simulink library "tqr"  (R2021b)
settings: Solver=VariableStepAuto  StartTime=0.0  StopTime=10.0  RelTol=1e-3
undefined symbols (not defined in the file or in its folder): ATQR_AltRDCActiveFEDUInc_X_pct, ATQR_AltRDCActiveFEDUInc_Y_enum, ATQR_AltRDCActiveFEDUTs_X_pct, ATQR_AltRDCActiveFEDUTs_Y_enum, ATQR_AltRDCActiveREDUInc_X_pct, ATQR_AltRDCActiveREDUInc_Y_enum, ATQR_AltRDCActiveREDUTs_X_pct, ATQR_AltRDCActiveREDUTs_Y_enum, ATQR_CreepFEDUTqIncSR_X_rpm, ATQR_CreepFEDUTqIncSR_Y_Nm, ATQR_CreepFEDUTs_X_rpm, ATQR_CreepFEDUTs_Y_Nm, ATQR_EcoTqFrIncGain_X_Nm, ATQR_EcoTqFrIncGain_Y_pct, ATQR_EcoTqRrIncGain_X_Nm, ATQR_EcoTqRrIncGain_Y_pct, ATQR_EL1FEDUTqDecSR_Y_Nm, ATQR_EL1FEDUTqIncSR_X_rpm, ATQR_EL1FEDUTqIncSR_Y_pct, ATQR_EL1FEDUTs_X_rpm, ATQR_EL1FEDUTs_Y_Nm, ATQR_EL1REDUTqDecSR_Y_Nm, ATQR_EL1REDUTs_Y_Nm, ATQR_FEDUEL1RegenTs_X_rpm, ATQR_FEDUTIPOutTs_X_rpm, ATQR_FrNegRateLimitIncN_X_rpm, ATQR_FrNegRateLimitIncN_Y_Nm, ATQR_FrPosRateLimitIncN_X_rpm, ATQR_FrPosRateLimitIncN_Y_Nm, ATQR_FShaftSpdTqLimCoe_X_rpm, ATQR_FTimerTqLimCoe_X_s, ATQR_FTqZeroTransUpBoundN_X_rpm, ATQR_NL1FEDUTqDecSR_Y_Nm, ATQR_NL1FEDUTqIncSR_X_rpm, ATQR_NL1FEDUTqIncSR_Y_pct, ATQR_NL1FEDUTs_X_rpm, ATQR_NL1FEDUTs_Y_Nm, ATQR_NL1REDUTqDecSR_Y_Nm, ATQR_NL1REDUTs_Y_Nm, ATQR_NormalTqFrIncGain_X_Nm, ATQR_NormalTqFrIncGain_Y_pct, ATQR_NormalTqRrIncGain_X_Nm, ATQR_NormalTqRrIncGain_Y_pct, ATQR_RrNegRateLimitIncN_X_rpm, ATQR_RrNegRateLimitIncN_Y_Nm, ATQR_RrPosRateLimitIncN_X_rpm, ATQR_RrPosRateLimitIncN_Y_Nm, ATQR_RShaftSpdTqLimCoe_X_rpm, ATQR_RTimerTqLimCoe_X_s, ATQR_SL1FEDUTqDecSR_Y_Nm, ATQR_SL1FEDUTqIncSR_X_rpm, ATQR_SL1FEDUTqIncSR_Y_pct, ATQR_SL1FEDUTs_X_rpm, ATQR_SL1FEDUTs_Y_Nm, ATQR_SL1REDUTqDecSR_Y_Nm, ATQR_SL1REDUTs_Y_Nm, ATQR_SportTqFrIncGain_X_Nm, ATQR_SportTqFrIncGain_Y_pct, ATQR_SportTqRrIncGain_X_Nm, ATQR_SportTqRrIncGain_Y_pct ... (+261)
libraries: hcu_lib x14, simulink x12, $bdroot x3
(part 2 of 9)

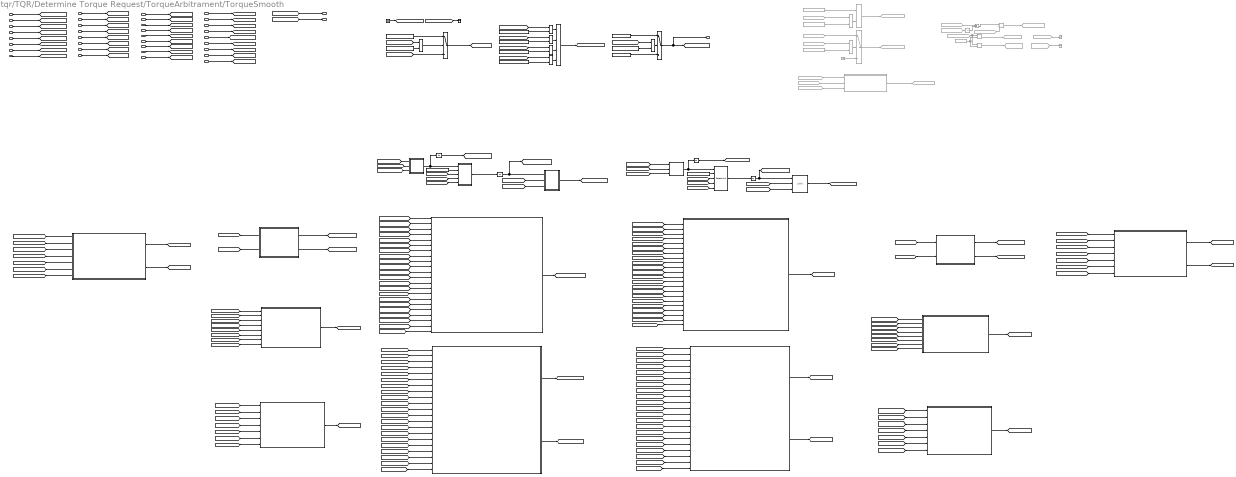
== system tqr/TQR/Determine Torque Request/TorqueArbitrament/TorqueSmooth ==
  note: Fr | Rr
  note: Front First order filter input tau map and determination
  note: Rear Rate limitation map and determination
  note: Front Rate limitation map and determination
  note: Rear wheel first order filter input torque command determination
  note: Front wheel first order filter input torque command determination:
  note: Rear Torque zero point transfer status determination
  note: Front Torque zero point transfer status determination
  note: Front Torque zero point transfer boundary map
  note: Rear Torque zero point transfer boundary map
  note: Rear First order filter input tau map and determination
  note: Rear torque ramp limtation and determination
  note: Rear torque ramp limtation and determination
  note: Rear Final Torque
  note: Front Final Torque
  task_time_s : Inport
  VDHP_ActAPSPosn_pct : Inport  Port=2
  VTQD_TqTargetShaftSpd_rpm : Inport  Port=3
  VTQD_TqSourceFr_enum : Inport  Port=4
  VTQD_TqSourceRr_enum : Inport  Port=5
  VTQD_AfterAvailableTqDemRr_Nm : Inport  Port=6
  VTQD_AfterAvailableTqDemFr_Nm : Inport  Port=7
  VTQD_EVDriveMode_enum : Inport  Port=8
  VTQD_EVDriveModeValid_flg : Inport  Port=9
  VTQD_RollRegenEnable_flg : Inport  Port=10
  VINP_VehSpeed_kph : Inport  Port=11
  VPMM_DriveTrainSelect_enum : Inport  Port=12
  VTQD_LimpHomeAct_flg : Inport  Port=13
  VTQD_RegenMode_enum : Inport  Port=14
  VVMC_ACCPedalOvrd_flg : Inport  Port=15
  VVMC_CCPedalOvrd_flg : Inport  Port=16
  VTQD_GearActualPosn_enum : Inport  Port=17
  VTQD_PreLoadHold_flg : Inport  Port=18
  VTQD_PreLoadPreEn_flg : Inport  Port=19
  VTQR_NoABSFEDUWhlTqReq_Nm : Inport  Port=20
  VTQR_NoABSREDUWhlTqReq_Nm : Inport  Port=21
  VTQD_CreepPrLoadEnable_flg : Inport  Port=22
  VVMC_ADASActive_flg : Inport  Port=23
  VTQD_RDCActive_enum : Inport  Port=24
  VVMC_ActMaxSlideRate_pct : Inport  Port=25
  VTQD_RegenTqLimitEn_flg : Inport  Port=26
  VTQD_PedAccTqEn_flg : Inport  Port=27
  VTQR_FrGearChange_flg : Inport  Port=28
  VTQR_RrGearChange_flg : Inport  Port=29
  VVMC_MSAWhlTqActive_flg : Inport  Port=30
  VINP_LFRawWhlSpeed_kph : Inport  Port=31
  VINP_RFRawWhlSpeed_kph : Inport  Port=32
  VINP_LRRawWhlSpeed_kph : Inport  Port=33
  VINP_RRRawWhlSpeed_kph : Inport  Port=34
  AND : Logic  Inputs=4  AllPortsSameDT=off  OutDataTypeStr=boolean
  AND18 : Logic  Commented=on  AllPortsSameDT=off  OutDataTypeStr=boolean
  Constant : Constant  Value=ZERO_FLOAT
  Constant1 : Constant  Value=ZERO_FLOAT
  Constant2 : Constant  Value=ENUM_REGENLEVEL_LV1
  Constant3 : Constant  Value=MINUSONE_FLOAT
  Constant36 : Constant  Commented=on  Value=KTQR_AWDSynchEnbl_flg
  Constant38 : Constant  Commented=on  Value=ENUM_DRIVETRAIN_AWD
  Constant4 : Constant  Value=ENUM_DRIVEMODE_SPORT
  Constant41 : Constant  Commented=on  Value=ZERO_INT
  Constant47 : Constant  Commented=on  Value=ENUM_DRIVETRAIN_FWD
  Constant5 : Constant  Value=KTQR_LaunchEnPedal_pct
  Constant6 : Constant  Value=KTQR_LaunchEnSpd_kph
  Constant7 : Constant  Value=ONE_FLOAT
  Divide : Product  Commented=on  Inputs=*/
  Equal{,1..3} (4 alike) : RelationalOperator  Operator===  OutDataTypeStr=boolean  RndMeth=Simplest
  Equal34 : RelationalOperator  Commented=on  Operator===  OutDataTypeStr=boolean  RndMeth=Simplest
  Equal35 : RelationalOperator  Commented=on  Operator===  OutDataTypeStr=boolean  RndMeth=Simplest
  FirstOrderFilter : Subsystem  RTWFileName=HCU_LIB  mask(FirstOrderFilter){}
      mask help: First order Filter.
      settings: RTWFileNameOpts=User specified
  FirstOrderFilter1 : $bdroot/TQR/Determine Torque Request/TorqueArbitrament/TorqueSmooth/FirstOrderFilter
  From125 : From  Commented=on  GotoTag=VDHP_ActAPSPosn_pct
  From127 : From  Commented=on  GotoTag=VTQR_ActAPSPosnAcc_enum
  From139 : From  Commented=on  GotoTag=VTQR_PedalAcc_flg
  From140 : From  Commented=on  GotoTag=VTQR_PedalDec_flg
  From141 : From  Commented=on  GotoTag=VDHP_ActAPSPosn_pct
  From142 : From  Commented=on  GotoTag=task_time_s
  From153 : From  Commented=on  GotoTag=VTQD_TqTargetShaftSpd_rpm
  From154 : From  Commented=on  GotoTag=VPMM_DriveTrainSelect_enum
  From155 : From  Commented=on  GotoTag=VPMM_DriveTrainSelect_enum
  From5 : From  Commented=on  GotoTag=VTQD_DRTransfer_flg
      settings: CloseFcn=tagdialog Close
  From6 : From  Commented=on  GotoTag=NTQR_TMTqReq_Nm
      settings: CloseFcn=tagdialog Close
  From9 : From  Commented=on  GotoTag=VTQR_TMTqReqLimit_Nm
      settings: CloseFcn=tagdialog Close
  Front First order filter input tau map and determination : Subsystem
  Front Torque zero point transfer boundary map : Subsystem
  "Front Torque zero point transfer status determination " : Subsystem
  Front torque ramp limtation and determination : Subsystem
  Front wheel first order filter input torque command determination : Subsystem
  Front wheel rate limit determination : Subsystem
  Goto19 : Goto  Commented=on  GotoTag=VTQR_AWDSynchEnbl_flg
  Goto2 : Goto  Commented=on  GotoTag=VTQR_ZeroTqRecover_flg
  Goto22 : Goto  Commented=on  GotoTag=VTQR_ActAPSPosnAcc_enum
  Goto23 : Goto  Commented=on  GotoTag=VTQR_PedalAcc_flg
  Goto24 : Goto  Commented=on  GotoTag=VTQR_PedalDec_flg
  Goto9 : Goto  Commented=on  GotoTag=VTQD_CAN2TqTargetShaftSpd_rpm
  GreaterThan : RelationalOperator  Commented=on  Operator=>  OutDataTypeStr=boolean  RndMeth=Simplest
  Ground : Ground  Commented=on
  Ground1 : Ground
  Less Than : RelationalOperator  Commented=on  Operator=<  OutDataTypeStr=boolean  RndMeth=Simplest
  Limit : Subsystem  RTWFileName=HCU_LIB  mask(Limit){}
      mask help: Limit funcion.
      settings: RTWFileNameOpts=User specified
  Limit2 : $bdroot/TQR/Determine Torque Request/TorqueArbitrament/TorqueSmooth/Limit
  RateLimit : Subsystem  RTWFileName=HCU_LIB  mask(RateLimit){}
      mask help: Rate limit function.
      settings: RTWFileNameOpts=User specified
  RateLimit1 : $bdroot/TQR/Determine Torque Request/TorqueArbitrament/TorqueSmooth/RateLimit
  Rear First order filter input tau map and determination : Subsystem
  Rear Torque zero point transfer boundary map : Subsystem
  "Rear Torque zero point transfer status determination " : Subsystem
  Rear torque ramp limtation and determination : Subsystem
  Rear wheel first order filter input torque command determination : Subsystem
  Rear wheel rate limit determination : Subsystem
  RegenLV_inc1 : Constant  Value=ENUM_GEARACTUALPOSN_R
  RegenLV_inc5 : Constant  Value=ENUM_GEARACTUALPOSN_R
  RegenLV_inc6 : Constant  Value=ENUM_DRIVEMODE_NRM
  Relational Operator4 : RelationalOperator  Operator=>  OutDataTypeStr=boolean  RndMeth=Simplest
  Relational Operator6 : RelationalOperator  Operator=<=  OutDataTypeStr=boolean  RndMeth=Simplest
  Subtract : Sum  Commented=on  Inputs=+-
  Switch : Switch  Criteria=u2 ~= 0
  Switch1 : Switch  Criteria=u2 > Threshold
  Switch10 : Switch  Commented=on  Criteria=u2 ~= 0
      settings: AttributesFormatString=<%<Criteria>>
  Terminator : Terminator  Commented=on
  Terminator1 : Terminator  Commented=on
  Terminator2 : Terminator
  Unit Delay : UnitDelay  Commented=on  SampleTime=-1  HasFrameUpgradeWarning=on
  Unit Delay{1..4} (4 alike) : UnitDelay  SampleTime=-1
  Zero Torque Revert : Subsystem  Commented=on
  VTQR_RampFEDUWhlTqReq_Nm : Outport
  VTQR_RampREDUWhlTqReq_Nm : Outport  Port=2
  VTQR_RampTqCMDGain_c : Outport  Port=3
  wires:
  [task_time_s] -> FirstOrderFilter/2(Tc)
  FirstOrderFilter/1(out) -> Unit Delay3/1, RateLimit/1(input_raw)  "VTQR_FrFirstOrderOutTq_Nm"
  task_time_s/1 -> [task_time_s]
  RateLimit/1(output) -> Unit Delay1/1  "VTQR_FEDUWhlTqReqSmooth_Nm"
  Unit Delay1/1 -> [VTQR_FEDUWhlTqReqSmoothDelay_Nm], Limit/1(input)  "VTQR_FEDUWhlTqReqSmoothDelay_Nm"
  From5/1 -> Zero Torque Revert/1(VTQD_DRTransfer_flg)
  Zero Torque Revert/1(VTQR_ZeroTqRecover_flg) -> Goto2/1
  From6/1 -> Zero Torque Revert/2(NTQR_TMTqReq_Nm)
  From9/1 -> Zero Torque Revert/3(VTQR_TMTqReqLimit_Nm)
  [VTQR_ActFEDUTrqUpLim_Nm] -> Limit/2(upper_limit)
  [VTQR_ActFEDUTrqLowLim_Nm] -> Limit/3(lower_limit)
  Limit/1(out) -> [VTQR_RampFEDUWhlTqReq_Nm]  "VTQR_RampFEDUWhlTqReq_Nm"
  [task_time_s] -> RateLimit/3(steptime)
  Constant/1 -> RateLimit/2(initial_value)
  VTQD_TqSourceFr_enum/1 -> [VTQD_TqSourceFr_enum]
  VDHP_ActAPSPosn_pct/1 -> [VDHP_ActAPSPosn_pct]
  VTQD_AfterAvailableTqDemFr_Nm/1 -> [VTQD_AfterAvailableTqDemFr_Nm]
  VTQD_AfterAvailableTqDemRr_Nm/1 -> [VTQD_AfterAvailableTqDemRr_Nm]
  Unit Delay2/1 -> [VTQR_REDUWhlTqReqSmoothDelay_Nm], Limit2/1  "VTQR_REDUWhlTqReqSmoothDelay_Nm"
  RateLimit1/1 -> Unit Delay2/1  "VTQR_REDUWhlTqReqSmooth_Nm"
  FirstOrderFilter1/1 -> Unit Delay4/1, RateLimit1/1  "VTQR_RrFirstOrderOutTq_Nm"
  [task_time_s] -> FirstOrderFilter1/2
  Limit2/1 -> [VTQR_RampREDUWhlTqReq_Nm]  "VTQR_RampREDUWhlTqReq_Nm"
  [task_time_s] -> RateLimit1/3
  Constant1/1 -> RateLimit1/2
  VTQD_EVDriveMode_enum/1 -> [VTQD_EVDriveMode_enum]
  Constant38/1 -> Equal34/2
  Equal34/1 -> AND18/2
  From154/1 -> Equal34/1
  Constant36/1 -> AND18/1
  AND18/1 -> Goto19/1  "VTQR_AWDSynchEnbl_flg"
  From125/1 -> Subtract/1
  Divide/1 -> Goto22/1  "VTQR_ActAPSPosnAcc_enum"
  From127/1 -> Less Than/1, GreaterThan/1
  Constant41/1 -> Less Than/2, GreaterThan/2
  GreaterThan/1 -> Goto23/1  "VTQR_PedalAcc_flg"
  Less Than/1 -> Goto24/1  "VTQR_PedalDec_flg"
  From139/1 -> Terminator/1
  From140/1 -> Terminator1/1
  From141/1 -> Unit Delay/1
  Unit Delay/1 -> Subtract/2
  Subtract/1 -> Divide/1
  From142/1 -> Divide/2
  VTQD_RollRegenEnable_flg/1 -> [VTQD_RollRegenEnable_flg]
  VINP_VehSpeed_kph/1 -> [VINP_VehSpeed_kph]
  From155/1 -> Equal35/1
  Constant47/1 -> Equal35/2
  Equal35/1 -> Switch10/2
  Switch10/1 -> Goto9/1
  From153/1 -> Switch10/1
  VPMM_DriveTrainSelect_enum/1 -> [VPMM_DriveTrainSelect_enum]
  VTQD_LimpHomeAct_flg/1 -> [VTQD_LimpHomeAct_flg]
  VTQD_EVDriveModeValid_flg/1 -> [VTQD_EVDriveModeValid_flg]
  Ground/1 -> Switch10/3
  VTQD_TqSourceRr_enum/1 -> [VTQD_TqSourceRr_enum]
  [VTQR_FEDUWhlTqReqSmoothDelay_Nm] -> "Front Torque zero point transfer status determination "/1(VTQR_FEDUWhlTqReqSmoothDelay_Nm)
  [VTQR_FrTqZeroTransUpBound_Nm] -> "Front Torque zero point transfer status determination "/2(VTQR_FrTqZeroTransUpBound_Nm)
  [VTQR_FrTqZeroTransLowBound_Nm] -> "Front Torque zero point transfer status determination "/3(VTQR_FrTqZeroTransLowBound_Nm)
  "Front Torque zero point transfer status determination "/1(VTQR_FrTqZeroTrans_enum) -> [VTQR_FrTqZeroTrans_enum]
  Front wheel first order filter input torque command determination/1(VTQR_FrFirstOrderInpTq_Nm) -> [VTQR_FrFirstOrderInpTq_Nm]
  Rear wheel first order filter input torque command determination/1(VTQR_RrFirstOrderInpTq_Nm) -> [VTQR_RrFirstOrderInpTq_Nm]
  [VTQR_FrTqZeroTrans_enum] -> Front wheel rate limit determination/1(VTQR_FrTqZeroTrans_enum)
  [VTQD_TqSourceFr_enum] -> Front wheel rate limit determination/2(VTQD_TqSourceFr_enum)
  [VTQD_TqTargetShaftSpd_rpm] -> Front wheel rate limit determination/3(VTQD_TqTargetShaftSpd_rpm)
  Front wheel rate limit determination/2(VTQR_FrRateLimitDec_Nm) -> [VTQR_FrRateLimitDec_Nm]
  Front wheel rate limit determination/1(VTQR_FrRateLimitInc_Nm) -> [VTQR_FrRateLimitInc_Nm]
  [VTQR_FrFirstOrderInpTq_Nm] -> FirstOrderFilter/1(in)
  [VTQR_RrFirstOrderInpTq_Nm] -> FirstOrderFilter1/1
  [VTQR_FrRateLimitInc_Nm] -> RateLimit/4(ratelimt_inc)
  [VTQR_FrRateLimitDec_Nm] -> RateLimit/5(ratelimt_dec)
  Rear wheel rate limit determination/1(VTQR_RrRateLimitInc_Nm) -> [VTQR_RrRateLimitInc_Nm]
  Rear wheel rate limit determination/2(VTQR_RrRateLimitDec_Nm) -> [VTQR_RrRateLimitDec_Nm]
  [VTQD_TqTargetShaftSpd_rpm] -> Rear wheel rate limit determination/3(VTQD_TqTargetShaftSpd_rpm)
  [VTQD_TqSourceRr_enum] -> Rear wheel rate limit determination/2(VTQD_TqSourceRr_enum)
  [VTQR_RrTqZeroTrans_enum] -> Rear wheel rate limit determination/1(VTQR_RrTqZeroTrans_enum)
  [VTQR_RrRateLimitInc_Nm] -> RateLimit1/4
  [VTQR_RrRateLimitDec_Nm] -> RateLimit1/5
  Unit Delay3/1 -> [VTQR_FrFirstOrderOutTqDelay_Nm]  "VTQR_FrFirstOrderOutTqDelay_Nm"
  Front First order filter input tau map and determination/1(VTQR_FrFirstOrderInpTs_c) -> [VTQR_FrFirstOrderInpTs_c]
  [VTQR_FrFirstOrderInpTs_c] -> FirstOrderFilter/3(Ts)
  Rear First order filter input tau map and determination/1(VTQR_RrFirstOrderInpTs_c) -> [VTQR_RrFirstOrderInpTs_c]
  [VTQR_RrFirstOrderInpTs_c] -> FirstOrderFilter1/3
  Unit Delay4/1 -> [VTQR_RrFirstOrderOutTqDelay_Nm]  "VTQR_RrFirstOrderOutTqDelay_Nm"
  [VTQD_TqTargetShaftSpd_rpm] -> Front First order filter input tau map and determination/1(VTQD_TqTargetShaftSpd_rpm)
  [VTQR_EVDriveMode_enum] -> Front First order filter input tau map and determination/2(VTQR_EVDriveMode_enum)
  [VTQD_RollRegenEnable_flg] -> Front First order filter input tau map and determination/3(VTQD_RollRegenEnable_flg)
  [VTQD_TqSourceFr_enum] -> Front First order filter input tau map and determination/4(VTQD_TqSourceFr_enum)
  [VTQR_FEDUWhlTqReqSmoothDelay_Nm] -> Front First order filter input tau map and determination/5(VTQR_FEDUWhlTqReqSmoothDelay_Nm)
  [VDHP_ActAPSPosn_pct] -> Front First order filter input tau map and determination/6(VDHP_ActAPSPosn_pct)
  [VINP_VehSpeed_kph] -> Front First order filter input tau map and determination/7(VINP_VehSpeed_kph)
  [VTQD_LimpHomeAct_flg] -> Front First order filter input tau map and determination/8(VTQD_LimpHomeAct_flg)
  [VTQD_TqTargetShaftSpd_rpm] -> Rear First order filter input tau map and determination/1(VTQD_TqTargetShaftSpd_rpm)
  [VTQR_EVDriveMode_enum] -> Rear First order filter input tau map and determination/2(VTQR_EVDriveMode_enum)
  [VTQD_RollRegenEnable_flg] -> Rear First order filter input tau map and determination/3(VTQD_RollRegenEnable_flg)
  [VTQD_TqSourceRr_enum] -> Rear First order filter input tau map and determination/4(VTQD_TqSourceRr_enum)
  [VTQR_REDUWhlTqReqSmoothDelay_Nm] -> Rear First order filter input tau map and determination/5(VTQR_REDUWhlTqReqSmooth_Nm)
  [VDHP_ActAPSPosn_pct] -> Rear First order filter input tau map and determination/6(VDHP_ActAPSPosn_pct)
  [VINP_VehSpeed_kph] -> Rear First order filter input tau map and determination/7(VINP_VehSpeed_kph)
  [VTQD_LimpHomeAct_flg] -> Rear First order filter input tau map and determination/8(VTQD_LimpHomeAct_flg)
  [VTQD_LimpHomeAct_flg] -> Front wheel rate limit determination/4(VTQD_LimpHomeAct_flg)
  [VTQR_EVDriveMode_enum] -> Front wheel rate limit determination/5(VTQR_EVDriveMode_enum)
  [VDHP_ActAPSPosn_pct] -> Front wheel rate limit determination/6(VDHP_ActAPSPosn_pct)
  [VTQR_FEDUWhlTqReqSmoothDelay_Nm] -> Front wheel rate limit determination/7(VTQR_FEDUWhlTqReqSmoothDelay_Nm)
  [VTQD_EVDriveModeValid_flg] -> Front wheel rate limit determination/8(VTQD_EVDriveModeValid_flg)
  [VTQD_LimpHomeAct_flg] -> Rear wheel rate limit determination/4(VTQD_LimpHomeAct_flg)
  [VTQR_EVDriveMode_enum] -> Rear wheel rate limit determination/5(VTQR_EVDriveMode_enum)
  [VDHP_ActAPSPosn_pct] -> Rear wheel rate limit determination/6(VDHP_ActAPSPosn_pct)
  [VTQR_REDUWhlTqReqSmoothDelay_Nm] -> Rear wheel rate limit determination/7(VTQR_REDUWhlTqReqSmoothDelay_Nm)
  [VTQD_EVDriveModeValid_flg] -> Rear wheel rate limit determination/8(VTQD_EVDriveModeValid_flg)
  [VTQD_EVDriveModeValid_flg] -> Rear First order filter input tau map and determination/9(VTQD_EVDriveModeValid_flg)
  [VTQD_EVDriveModeValid_flg] -> Front First order filter input tau map and determination/9(VTQD_EVDriveModeValid_flg)
  [VTQD_TqTargetShaftSpd_rpm] -> Front Torque zero point transfer boundary map/1(VTQD_TqTargetShaftSpd_rpm)
  [VTQR_EVDriveMode_enum] -> Front Torque zero point transfer boundary map/2(VTQR_EVDriveMode_enum)
  Front Torque zero point transfer boundary map/1(VTQR_FrTqZeroTransUpBound_Nm) -> [VTQR_FrTqZeroTransUpBound_Nm]
  Front Torque zero point transfer boundary map/2(VTQR_FrTqZeroTransLowBound_Nm) -> [VTQR_FrTqZeroTransLowBound_Nm]
  [VTQD_TqTargetShaftSpd_rpm] -> Rear Torque zero point transfer boundary map/1(VTQD_TqTargetShaftSpd_rpm)
  [VTQR_EVDriveMode_enum] -> Rear Torque zero point transfer boundary map/2(VTQR_EVDriveMode_enum)
  Rear Torque zero point transfer boundary map/1(VTQR_RrTqZeroTransUpBound_Nm) -> [VTQR_RrTqZeroTransUpBound_Nm]
  Rear Torque zero point transfer boundary map/2(VTQR_RrTqZeroTransLowBound_Nm) -> [VTQR_RrTqZeroTransLowBound_Nm]
  [VTQD_RegenMode_enum] -> Front First order filter input tau map and determination/10(VTQD_RegenMode_enum)
  VTQD_RegenMode_enum/1 -> [VTQD_RegenMode_enum]
  [VTQD_RegenMode_enum] -> Front wheel rate limit determination/9(VTQD_RegenMode_enum)
  [VTQD_RegenMode_enum] -> Rear First order filter input tau map and determination/10(VTQD_RegenMode_enum)
  [VTQD_RegenMode_enum] -> Rear wheel rate limit determination/9(VTQD_RegenMode_enum)
  VVMC_ACCPedalOvrd_flg/1 -> [VVMC_ACCPedalOvrd_flg]
  VVMC_CCPedalOvrd_flg/1 -> [VVMC_CCPedalOvrd_flg]
  RegenLV_inc5/1 -> Equal/2
  Equal/1 -> Switch/2
  RegenLV_inc6/1 -> Switch/1
  Switch/1 -> [VTQR_EVDriveMode_enum]  "VTQR_EVDriveMode_enum"
  [VTQD_GearActualPosn_enum] -> Equal/1
  [VTQD_EVDriveMode_enum] -> Switch/3
  VTQD_GearActualPosn_enum/1 -> [VTQD_GearActualPosn_enum]
  [VVMC_ACCPedalOvrd_flg] -> Front First order filter input tau map and determination/11(VVMC_ACCPedalOvrd_flg)
  [VVMC_CCPedalOvrd_flg] -> Front First order filter input tau map and determination/12(VVMC_CCPedalOvrd_flg)
  [VVMC_ACCPedalOvrd_flg] -> Front wheel rate limit determination/10(VVMC_ACCPedalOvrd_flg)
  [VVMC_CCPedalOvrd_flg] -> Front wheel rate limit determination/11(VVMC_CCPedalOvrd_flg)
  [VVMC_ACCPedalOvrd_flg] -> Rear First order filter input tau map and determination/11(VVMC_ACCPedalOvrd_flg)
  [VVMC_CCPedalOvrd_flg] -> Rear First order filter input tau map and determination/12(VVMC_CCPedalOvrd_flg)
  [VVMC_ACCPedalOvrd_flg] -> Rear wheel rate limit determination/10(VVMC_ACCPedalOvrd_flg)
  [VVMC_CCPedalOvrd_flg] -> Rear wheel rate limit determination/11(VVMC_CCPedalOvrd_flg)
  VTQD_TqTargetShaftSpd_rpm/1 -> [VTQD_TqTargetShaftSpd_rpm]
  VTQD_PreLoadHold_flg/1 -> [VTQD_PreLoadHold_flg]
  VTQD_PreLoadPreEn_flg/1 -> [VTQD_PreLoadPreEn_flg]
  [VTQD_PreLoadHold_flg] -> Rear First order filter input tau map and determination/13(VTQD_PreLoadHold_flg)
  [VTQD_PreLoadHold_flg] -> Front First order filter input tau map and determination/13(VTQD_PreLoadHold_flg)
  VTQR_NoABSFEDUWhlTqReq_Nm/1 -> [VTQR_NoABSFEDUWhlTqReq_Nm]
  VTQR_NoABSREDUWhlTqReq_Nm/1 -> [VTQR_NoABSREDUWhlTqReq_Nm]
  VTQD_CreepPrLoadEnable_flg/1 -> [VTQD_CreepPrLoadEnable_flg]
  VVMC_ADASActive_flg/1 -> [VVMC_ADASActive_flg]
  [VTQD_CreepPrLoadEnable_flg] -> "Front Torque zero point transfer status determination "/4(VTQD_CreepPrLoadEnable_flg)
  [VVMC_ADASActive_flg] -> "Front Torque zero point transfer status determination "/5(VVMC_ADASActive_flg)
  [VTQD_PreLoadPreEn_flg] -> "Front Torque zero point transfer status determination "/6(VTQD_PreLoadPreEn_flg)
  [VTQD_CreepPrLoadEnable_flg] -> Front First order filter input tau map and determination/15(VTQD_CreepPrLoadEnable_flg)
  [VTQD_CreepPrLoadEnable_flg] -> Rear First order filter input tau map and determination/15(VTQD_CreepPrLoadEnable_flg)
  [VTQD_CreepPrLoadEnable_flg] -> Front wheel rate limit determination/12(VTQD_CreepPrLoadEnable_flg)
  [VTQD_RDCActive_enum] -> Front wheel rate limit determination/14(VTQD_RDCActive_enum)
  [VTQD_PreLoadPreEn_flg] -> Front wheel rate limit determination/15(VTQD_PreLoadPreEn_flg)
  VTQD_RDCActive_enum/1 -> [VTQD_RDCActive_enum]
  [VTQD_PreLoadPreEn_flg] -> Rear wheel rate limit determination/15(VTQD_PreLoadPreEn_flg)
  [VTQD_CreepPrLoadEnable_flg] -> Rear wheel rate limit determination/12(VTQD_CreepPrLoadEnable_flg)
  [VTQD_RDCActive_enum] -> Rear wheel rate limit determination/14(VTQD_RDCActive_enum)
  Ground1/1 -> [VINP_SCPSystemMode_enum]
  [VTQD_RDCActive_enum] -> Front First order filter input tau map and determination/16(VTQD_RDCActive_enum)
  [VTQR_NoABSFEDUWhlTqReq_Nm] -> Front First order filter input tau map and determination/17(VTQR_NoABSFEDUWhlTqReq_Nm)
  [VTQR_RampFEDUWhlTqReq_Nm] -> Front First order filter input tau map and determination/18(VTQR_RampFEDUWhlTqReq_Nm)
  [VTQR_NoABSFEDUWhlTqReq_Nm] -> Front wheel rate limit determination/16(VTQR_NoABSFEDUWhlTqReq_Nm)
  [VTQR_RampFEDUWhlTqReq_Nm] -> Front wheel rate limit determination/17(VTQR_RampFEDUWhlTqReq_Nm)
  [VTQD_RDCActive_enum] -> Rear First order filter input tau map and determination/16(VTQD_RDCActive_enum)
  [VTQR_NoABSREDUWhlTqReq_Nm] -> Rear First order filter input tau map and determination/17(VTQR_NoABSREDUWhlTqReq_Nm)
  [VTQR_RampREDUWhlTqReq_Nm] -> Rear First order filter input tau map and determination/18(VTQR_RampREDUWhlTqReq_Nm)
  [VTQR_NoABSREDUWhlTqReq_Nm] -> Rear wheel rate limit determination/16(VTQR_NoABSREDUWhlTqReq_Nm)
  [VTQR_RampREDUWhlTqReq_Nm] -> Rear wheel rate limit determination/17(VTQR_RampREDUWhlTqReq_Nm)
  [VTQR_FrFirstOrderInpTq_Nm] -> Front First order filter input tau map and determination/19(VTQR_FrFirstOrderInpTq_Nm)
  [VTQR_FrFirstOrderInpTq_Nm] -> Front wheel rate limit determination/18(VTQR_FrFirstOrderInpTq_Nm)
  [VTQR_RrFirstOrderInpTq_Nm] -> Rear First order filter input tau map and determination/19(VTQR_RrFirstOrderInpTq_Nm)
  [VTQR_RrFirstOrderInpTq_Nm] -> Rear wheel rate limit determination/18(VTQR_RrFirstOrderInpTq_Nm)
  [VTQR_ActREDUTrqUpLim_Nm] -> Limit2/2
  [VTQR_ActREDUTrqLowLim_Nm] -> Limit2/3
  VVMC_ActMaxSlideRate_pct/1 -> [VVMC_ActMaxSlideRate_pct]
  VTQD_RegenTqLimitEn_flg/1 -> [VTQD_RegenTqLimitEn_flg]
  VTQD_PedAccTqEn_flg/1 -> [VTQD_PedAccTqEn_flg]
  [VVMC_ActMaxSlideRate_pct] -> Front First order filter input tau map and determination/14(VVMC_ActMaxSlideRate_pct)
  [VVMC_ActMaxSlideRate_pct] -> Front wheel rate limit determination/19(VVMC_ActMaxSlideRate_pct)
  [VTQD_PedAccTqEn_flg] -> Front wheel rate limit determination/20(VTQD_PedAccTqEn_flg)
  [VTQD_RegenTqLimitEn_flg] -> Front wheel rate limit determination/13(VTQD_RegenTqLimitEn_flg)
  [VTQD_PedAccTqEn_flg] -> Rear wheel rate limit determination/20(VTQD_PedAccTqEn_flg)
  [VVMC_ActMaxSlideRate_pct] -> Rear wheel rate limit determination/19(VVMC_ActMaxSlideRate_pct)
  [VVMC_ActMaxSlideRate_pct] -> Rear First order filter input tau map and determination/14(VVMC_ActMaxSlideRate_pct)
  [VTQD_PedAccTqEn_flg] -> Rear First order filter input tau map and determination/20(VTQD_PedAccTqEn_flg)
  Constant5/1 -> Relational Operator4/2
  Relational Operator4/1 -> AND/1
  Equal2/1 -> AND/4
  [VTQR_EVDriveMode_enum] -> Equal1/1
  Equal1/1 -> AND/3
  [VDHP_ActAPSPosn_pct] -> Relational Operator4/1
  [VINP_VehSpeed_kph] -> Relational Operator6/1
  Relational Operator6/1 -> AND/2
  AND/1 -> [VTQR_LaunchEn_flg]  "VTQR_LaunchEn_flg"
  [VTQD_RegenMode_enum] -> Equal2/1
  Constant6/1 -> Relational Operator6/2
  Constant2/1 -> Equal2/2
  Constant4/1 -> Equal1/2
  [VTQR_LaunchEn_flg] -> "Front Torque zero point transfer status determination "/7(VTQR_LaunchEn_flg)
  [VVMC_ACCPedalOvrd_flg] -> "Front Torque zero point transfer status determination "/8(VVMC_ACCPedalOvrd_flg)
  [VTQR_LaunchEn_flg] -> "Rear Torque zero point transfer status determination "/7(VTQR_LaunchEn_flg)
  [VTQD_CreepPrLoadEnable_flg] -> "Rear Torque zero point transfer status determination "/4(VTQD_CreepPrLoadEnable_flg)
  "Rear Torque zero point transfer status determination "/1(VTQR_RrTqZeroTrans_enum) -> [VTQR_RrTqZeroTrans_enum]
  [VVMC_ADASActive_flg] -> "Rear Torque zero point transfer status determination "/5(VVMC_ADASActive_flg)
  [VTQD_PreLoadPreEn_flg] -> "Rear Torque zero point transfer status determination "/6(VTQD_PreLoadPreEn_flg)
  [VTQR_REDUWhlTqReqSmoothDelay_Nm] -> "Rear Torque zero point transfer status determination "/1(VTQR_REDUWhlTqReqSmoothDelay_Nm)
  [VVMC_ACCPedalOvrd_flg] -> "Rear Torque zero point transfer status determination "/8(VVMC_ACCPedalOvrd_flg)
  [VTQR_RrTqZeroTransLowBound_Nm] -> "Rear Torque zero point transfer status determination "/3(VTQR_RrTqZeroTransLowBound_Nm)
  [VTQR_RrTqZeroTransUpBound_Nm] -> "Rear Torque zero point transfer status determination "/2(VTQR_RrTqZeroTransUpBound_Nm)
  [VTQD_PedAccTqEn_flg] -> Front First order filter input tau map and determination/20(VTQD_PedAccTqEn_flg)
  [VTQD_RegenTqLimitEn_flg] -> Rear wheel rate limit determination/13(VTQD_RegenTqLimitEn_flg)
  [VTQR_RampFEDUWhlTqReq_Nm] -> VTQR_RampFEDUWhlTqReq_Nm/1  "VTQR_RampFEDUWhlTqReq_Nm"
  [VTQR_RampREDUWhlTqReq_Nm] -> VTQR_RampREDUWhlTqReq_Nm/1  "VTQR_RampREDUWhlTqReq_Nm"
  [VTQR_FrGearChange_flg] -> Front wheel first order filter input torque command determination/6(VTQR_FrGearChange_flg)
  [VTQR_FrFirstOrderOutTqDelay_Nm] -> Front wheel first order filter input torque command determination/5(VTQR_FrFirstOrderOutTqDelay_Nm)
  [VTQR_FrTqZeroTrans_enum] -> Front wheel first order filter input torque command determination/1(VTQR_FrTqZeroTrans_enum)
  [VTQD_AfterAvailableTqDemFr_Nm] -> Front wheel first order filter input torque command determination/4(VTQD_AfterAvailableTqDemFr_Nm)
  [VTQR_FrTqZeroTransLowBound_Nm] -> Front wheel first order filter input torque command determination/3(VTQR_FrTqZeroTransLowBound_Nm)
  [VTQR_FrTqZeroTransUpBound_Nm] -> Front wheel first order filter input torque command determination/2(VTQR_FrTqZeroTransUpBound_Nm)
  [VTQR_RrGearChange_flg] -> Rear wheel first order filter input torque command determination/6(VTQR_RrGearChange_flg)
  [VTQR_RrTqZeroTransUpBound_Nm] -> Rear wheel first order filter input torque command determination/2(VTQR_RrTqZeroTransUpBound_Nm)
  [VTQD_AfterAvailableTqDemRr_Nm] -> Rear wheel first order filter input torque command determination/4(VTQD_AfterAvailableTqDemRr_Nm)
  [VTQR_RrTqZeroTransLowBound_Nm] -> Rear wheel first order filter input torque command determination/3(VTQR_RrTqZeroTransLowBound_Nm)
  [VTQR_RrFirstOrderOutTqDelay_Nm] -> Rear wheel first order filter input torque command determination/5(VTQR_RrFirstOrderOutTqDelay_Nm)
  [VTQR_RrTqZeroTrans_enum] -> Rear wheel first order filter input torque command determination/1(VTQR_RrTqZeroTrans_enum)
  VTQR_RrGearChange_flg/1 -> [VTQR_RrGearChange_flg]
  VTQR_FrGearChange_flg/1 -> [VTQR_FrGearChange_flg]
  [VINP_SCPSystemMode_enum] -> Terminator2/1
  [VTQD_PreLoadPreEn_flg] -> Front First order filter input tau map and determination/21(VTQD_PreLoadPreEn_flg)
  [VTQD_PreLoadPreEn_flg] -> Rear First order filter input tau map and determination/21(VTQD_PreLoadPreEn_flg)
  RegenLV_inc1/1 -> Equal3/2
  Equal3/1 -> Switch1/2
  [VTQD_GearActualPosn_enum] -> Equal3/1
  Constant3/1 -> Switch1/1
  Constant7/1 -> Switch1/3
  Switch1/1 -> VTQR_RampTqCMDGain_c/1, [VTQR_RampTqCMDGain_c]  "VTQR_RampTqCMDGain_c"
  [VTQR_RampTqCMDGain_c] -> Front wheel first order filter input torque command determination/7(VTQR_RampTqCMDGain_c)
  [VTQR_RampTqCMDGain_c] -> Rear wheel first order filter input torque command determination/7(VTQR_RampTqCMDGain_c)
  VVMC_MSAWhlTqActive_flg/1 -> [VVMC_MSAWhlTqActive_flg]
  [VVMC_MSAWhlTqActive_flg] -> Front First order filter input tau map and determination/22(VVMC_MSAWhlTqActive_flg)
  [VVMC_MSAWhlTqActive_flg] -> Front wheel rate limit determination/21(VVMC_MSAWhlTqActive_flg)
  [VVMC_MSAWhlTqActive_flg] -> Rear First order filter input tau map and determination/22(VVMC_MSAWhlTqActive_flg)
  [VVMC_MSAWhlTqActive_flg] -> Rear wheel rate limit determination/21(VVMC_MSAWhlTqActive_flg)
  [task_time_s] -> Front torque ramp limtation and determination/7(task_time_s)
  [VTQR_REDUWhlTqReqSmoothDelay_Nm] -> Front torque ramp limtation and determination/3(VTQR_REDUWhlTqReqSmoothDelay_Nm)
  [VINP_RFRawWhlSpeed_kph] -> Front torque ramp limtation and determination/6(VINP_RFRawWhlSpeed_kph)
  [VTQD_AfterAvailableTqDemFr_Nm] -> Front torque ramp limtation and determination/1(VTQD_AfterAvailableTqDemFr_Nm)
  Front torque ramp limtation and determination/2(VTQR_ActFEDUTrqLowLim_Nm) -> [VTQR_ActFEDUTrqLowLim_Nm]
  [VPMM_DriveTrainSelect_enum] -> Front torque ramp limtation and determination/4(VPMM_DriveTrainSelect_enum)
  [VTQD_AfterAvailableTqDemRr_Nm] -> Front torque ramp limtation and determination/2(VTQD_AfterAvailableTqDemRr_Nm)
  Front torque ramp limtation and determination/1(VTQR_ActFEDUTrqUpLim_Nm) -> [VTQR_ActFEDUTrqUpLim_Nm]
  [VINP_LFRawWhlSpeed_kph] -> Front torque ramp limtation and determination/5(VINP_LFRawWhlSpeed_kph)
  [task_time_s] -> Rear torque ramp limtation and determination/7(task_time_s)
  [VINP_LRRawWhlSpeed_kph] -> Rear torque ramp limtation and determination/5(VINP_LRRawWhlSpeed_kph)
  [VINP_RRRawWhlSpeed_kph] -> Rear torque ramp limtation and determination/6(VINP_RRRawWhlSpeed_kph)
  [VPMM_DriveTrainSelect_enum] -> Rear torque ramp limtation and determination/4(VPMM_DriveTrainSelect_enum)
  [VTQR_FEDUWhlTqReqSmoothDelay_Nm] -> Rear torque ramp limtation and determination/3(VTQR_FEDUWhlTqReqSmoothDelay_Nm)
  [VTQD_AfterAvailableTqDemFr_Nm] -> Rear torque ramp limtation and determination/1(VTQD_AfterAvailableTqDemFr_Nm)
  Rear torque ramp limtation and determination/2(VTQR_ActREDUTrqLowLim_Nm) -> [VTQR_ActREDUTrqLowLim_Nm]
  [VTQD_AfterAvailableTqDemRr_Nm] -> Rear torque ramp limtation and determination/2(VTQD_AfterAvailableTqDemRr_Nm)
  Rear torque ramp limtation and determination/1(VTQR_ActREDUTrqUpLim_Nm) -> [VTQR_ActREDUTrqUpLim_Nm]
  VINP_LFRawWhlSpeed_kph/1 -> [VINP_LFRawWhlSpeed_kph]
  VINP_LRRawWhlSpeed_kph/1 -> [VINP_LRRawWhlSpeed_kph]
  VINP_RRRawWhlSpeed_kph/1 -> [VINP_RRRawWhlSpeed_kph]
  VINP_RFRawWhlSpeed_kph/1 -> [VINP_RFRawWhlSpeed_kph]

== system tqr/TQR/Determine Torque Request/TorqueArbitrament/TorqueSmooth/FirstOrderFilter ==
  in : Inport
  Tc : Inport  Port=2
  Ts : Inport  Port=3
  Add : Sum
  Add2 : Sum  Inputs=+-
  Constant3 : Constant  OutDataTypeStr=single
  Constant4 : Constant  Value=0  OutDataTypeStr=single
  Constant5 : Constant  Value=0  OutDataTypeStr=single
  Constant6 : Constant  Value=eps  OutDataTypeStr=single
  Divide : Product  Inputs=*/
  MinMax{1..4} (4 alike) : MinMax  Function=max  Inputs=2
  Product : Product  RndMeth=Zero
  Product1 : Product  RndMeth=Zero
  Unit Delay : UnitDelay  SampleTime=-1  HasFrameUpgradeWarning=on
  out : Outport
  wires:
  Add/1 -> out/1, Unit Delay/1
  Divide/1 -> Product1/1, Add2/2
  Constant3/1 -> Add2/1
  Add2/1 -> Product/2
  Product/1 -> Add/1
  Unit Delay/1 -> Product/1
  in/1 -> Product1/2
  Product1/1 -> Add/2
  Tc/1 -> MinMax2/1
  Constant4/1 -> MinMax2/2
  Ts/1 -> MinMax3/1
  Constant5/1 -> MinMax3/2
  MinMax3/1 -> MinMax1/2
  MinMax2/1 -> Divide/1, MinMax1/1
  MinMax1/1 -> MinMax4/1
  Constant6/1 -> MinMax4/2
  MinMax4/1 -> Divide/2

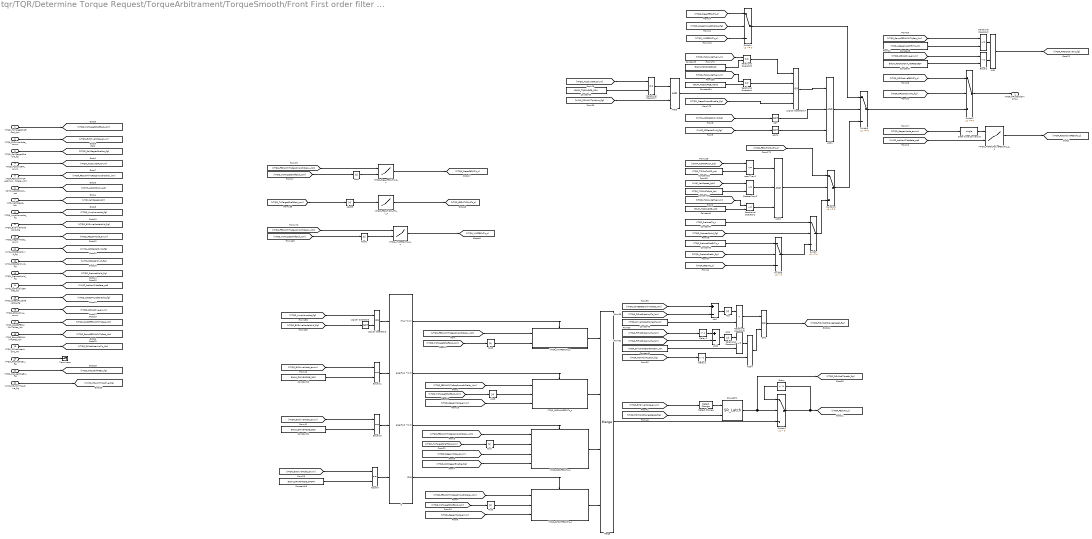
== system tqr/TQR/Determine Torque Request/TorqueArbitrament/TorqueSmooth/Front First order filter input tau map and determination ==
  VTQD_TqTargetShaftSpd_rpm : Inport
  VTQR_EVDriveMode_enum : Inport  Port=2
  VTQD_RollRegenEnable_flg : Inport  Port=3
  VTQD_TqSourceFr_enum : Inport  Port=4
  VTQR_FEDUWhlTqReqSmoothDelay_Nm : Inport  Port=5
  VDHP_ActAPSPosn_pct : Inport  Port=6
  VINP_VehSpeed_kph : Inport  Port=7
  VTQD_LimpHomeAct_flg : Inport  Port=8
  VTQD_EVDriveModeValid_flg : Inport  Port=9
  VTQD_RegenMode_enum : Inport  Port=10
  VVMC_ACCPedalOvrd_flg : Inport  Port=11
  VVMC_CCPedalOvrd_flg : Inport  Port=12
  VTQD_PreLoadHold_flg : Inport  Port=13
  VVMC_ActMaxSlideRate_pct : Inport  Port=14
  VTQD_CreepPrLoadEnable_flg : Inport  Port=15
  VTQD_RDCActive_enum : Inport  Port=16
  VTQR_NoABSFEDUWhlTqReq_Nm : Inport  Port=17
  VTQR_RampFEDUWhlTqReq_Nm : Inport  Port=18
  VTQR_FrFirstOrderInpTq_Nm : Inport  Port=19
  VTQD_PedAccTqEn_flg : Inport  Port=20
  VTQD_PreLoadPreEn_flg : Inport  Port=21
  VVMC_MSAWhlTqActive_flg : Inport  Port=22
  AND : Logic  AllPortsSameDT=off  OutDataTypeStr=boolean
  AND1 : Logic  Inputs=3  AllPortsSameDT=off  OutDataTypeStr=boolean
  AND2 : Logic  Inputs=3  AllPortsSameDT=off  OutDataTypeStr=boolean
  AND3 : Logic  AllPortsSameDT=off  OutDataTypeStr=boolean
  AND4 : Logic  AllPortsSameDT=off  OutDataTypeStr=boolean
  Abs{,1,4..8,38,41} (9 alike) : Abs
  Add : Sum  Inputs=+-
  Add1 : Sum  Inputs=+-
  Constant1 : Constant  Value=ENUM_TQSOURCE_APS
  Constant11 : Constant  Value=ENUM_DRIVEMODE_ECO
  Constant12 : Constant  Value=ENUM_DRIVEMODE_NRM
  Constant16 : Constant  Value=ENUM_DRIVEMODE_SPORT
  Constant2 : Constant  Value=KTQR_DriveModeCMDTqDev_Nm
  Constant3 : Constant  Value=ENUM_TQSOURCE_CC
  Constant32 : Constant  Value=KTQR_TIPOutTsAPS_pct
  Constant33 : Constant  Value=KTQR_TIPOutTsSpd_kph
  Constant34 : Constant  Value=ENUM_TQSOURCE_ADAS
  Constant4 : Constant  Value=KTQR_PreLoadTs_c
  Constant5 : Constant  Value=KTQR_ARegenLatchEnTq_Nm
  Constant6 : Constant  Value=KTQR_PreLoadPreEnTs_c
  Constant7 : Constant  Value=ENUM_RDCACTSTA_NOREQUEST
  Constant8 : Constant  Value=KTQR_DriveModeChangeTq_Nm
  Constant9 : Constant  Value=ENUM_TQSOURCE_MSA
  Data Type Conversion : DataTypeConversion  OutDataTypeStr=single
  Delay : Delay  DelayLength=1
  Delay1 : Delay  DelayLength=1
  Delay2 : Delay  DelayLength=1
  Detect Change : simulink/Logic and Bit Operations/Detect Change  vinit=0  OutDataTypeStr=boolean
  Equal10 : RelationalOperator  Operator===  OutDataTypeStr=boolean  RndMeth=Simplest
  Equal11 : RelationalOperator  Operator===  OutDataTypeStr=boolean  RndMeth=Simplest
  Equal2 : RelationalOperator  Operator=~=  OutDataTypeStr=boolean  RndMeth=Simplest
  Equal9 : RelationalOperator  Operator===  OutDataTypeStr=boolean  RndMeth=Simplest
  GreaterThan2 : RelationalOperator  OutDataTypeStr=boolean  RndMeth=Simplest
  If : If  NumInputs=4  IfExpression=u1~= 0  ElseIfExpressions=u2 ~= 0, u3 ~= 0
  Less Than2 : RelationalOperator  Operator=<=  OutDataTypeStr=boolean  RndMeth=Simplest
  Logical Operator14 : Logic  Operator=OR  Inputs=4  AllPortsSameDT=off  OutDataTypeStr=boolean
  Logical Operator2 : Logic  Operator=OR  AllPortsSameDT=off  OutDataTypeStr=boolean
  Logical Operator3 : Logic  Operator=NOT  AllPortsSameDT=off  OutDataTypeStr=boolean
  MTQR_AltRDCActiveFEDUTs_Z_c : Lookup_n-D  BreakpointsForDimension1=ATQR_AltRDCActiveFEDUTs_Y_enum  BreakpointsForDimension2=ATQR_AltRDCActiveFEDUTs_X_pct  Table=MTQR_AltRDCActiveFEDUTs_Z_c  TableDataTypeStr=Inherit: Inherit from 'Table data'  ExtrapMethod=Clip  InternalRulePriority=Speed  RndMeth=Simplest  InputSameDT=on
      settings: InputPortMap=u0,u1
  MTQR_CreepFEDUTs_Z_c : Lookup_n-D  BreakpointsForDimension1=ATQR_CreepFEDUTs_Y_Nm  BreakpointsForDimension2=ATQR_CreepFEDUTs_X_rpm  Table=MTQR_CreepFEDUTs_Z_c  ExtrapMethod=Clip  InternalRulePriority=Speed  RndMeth=Simplest  InputSameDT=on
      settings: InputPortMap=u0,u1
  MTQR_FEDUTIPOutTs_Y_c : Lookup_n-D  NumberOfTableDimensions=1  BreakpointsForDimension1=ATQR_FEDUTIPOutTs_X_rpm  Table=MTQR_FEDUTIPOutTs_Y_c  ExtrapMethod=Clip  InternalRulePriority=Speed  RndMeth=Simplest  InputSameDT=on
  MTQR_VMCFEDUTs_Z_c : Lookup_n-D  BreakpointsForDimension1=ATQR_VMCFEDUTs_Y_Nm  BreakpointsForDimension2=ATQR_VMCFEDUTs_X_rpm  Table=MTQR_VMCFEDUTs_Z_c  ExtrapMethod=Clip  InternalRulePriority=Speed  RndMeth=Simplest  InputSameDT=on
      settings: InputPortMap=u0,u1
  Merge : Merge  Inputs=4
  NOT : Logic  Operator=NOT  AllPortsSameDT=off  OutDataTypeStr=boolean
  NOT1 : Logic  Operator=NOT  AllPortsSameDT=off  OutDataTypeStr=boolean
  OR2 : Logic  Operator=OR  AllPortsSameDT=off  OutDataTypeStr=boolean
  Relational Operator1 : RelationalOperator  Operator=~=  OutDataTypeStr=boolean  RndMeth=Simplest
  Relational Operator2 : RelationalOperator  Operator=<=  OutDataTypeStr=boolean  RndMeth=Simplest
  Relational Operator3 : RelationalOperator  Operator===  OutDataTypeStr=boolean  RndMeth=Simplest
  Relational Operator4 : RelationalOperator  Operator===  OutDataTypeStr=boolean  RndMeth=Simplest
  Relational Operator5 : RelationalOperator  Operator=<  OutDataTypeStr=boolean  RndMeth=Simplest
  Relational Operator6 : RelationalOperator  OutDataTypeStr=boolean  RndMeth=Simplest
  Relational Operator7 : RelationalOperator  Operator===  OutDataTypeStr=boolean  RndMeth=Simplest
  SR_Latch1 : hcu_lib/Basic_Blocks/SR_Latch
  Switch : Switch  Criteria=u2 ~= 0
  Switch1 : Switch  Criteria=u2 ~= 0  Threshold=0.5
  Switch13 : Switch  Criteria=u2 ~= 0
  Switch2 : Switch  Criteria=u2 ~= 0
  Switch3 : Switch  Criteria=u2 ~= 0  Threshold=0.5
  Switch4 : Switch  Criteria=u2 > Threshold
  Switch5 : Switch  Criteria=u2 > Threshold
  Terminator : Terminator
  VTQR_ECOFEDUTs_c : Subsystem  TreatAsAtomicUnit=on
  VTQR_LHMFEDUTs_c : Subsystem  AncestorBlock=tqr_20221220/TQR/Determine Torque Request/TorqueArbitrament/TorqueSmooth/VTQR_LHMFEDUTs_c  TreatAsAtomicUnit=on
  VTQR_NORMALFEDUTs_c : Subsystem  TreatAsAtomicUnit=on
  VTQR_SPORTFEDUTs_c : Subsystem  AncestorBlock=tqr_20221220/TQR/Determine Torque Request/TorqueArbitrament/TorqueSmooth/VTQR_SPORTFEDUTs_c  TreatAsAtomicUnit=on
  VTQR_FrFirstOrderInpTs_c : Outport
  wires:
  Abs38/1 -> MTQR_FEDUTIPOutTs_Y_c/1
  MTQR_FEDUTIPOutTs_Y_c/1 -> [VTQR_FEDUTIPOutTs_c]  "VTQR_FEDUTIPOutTs_c"
  [VTQD_TqTargetShaftSpd_rpm] -> Abs38/1
  MTQR_VMCFEDUTs_Z_c/1 -> [VTQR_VMCFEDUTs_c]  "VTQR_VMCFEDUTs_c"
  [VTQD_TqTargetShaftSpd_rpm] -> Abs41/1
  Equal9/1 -> If/4
  Constant11/1 -> Equal10/2
  [VTQD_TqTargetShaftSpd_rpm] -> Abs6/1
  [VTQD_TqTargetShaftSpd_rpm] -> Abs8/1
  [VTQD_EVDriveModeValid_flg] -> Logical Operator3/1
  Constant12/1 -> Equal11/2
  [VTQR_EVDriveMode_enum] -> Equal11/1
  Constant16/1 -> Equal9/2
  [VTQR_EVDriveMode_enum] -> Equal10/1
  Logical Operator2/1 -> If/1
  [VTQD_LimpHomeAct_flg] -> Logical Operator2/1
  [VTQD_TqTargetShaftSpd_rpm] -> Abs5/1
  Equal10/1 -> If/3
  [VTQR_EVDriveMode_enum] -> Equal9/1
  [VTQD_TqTargetShaftSpd_rpm] -> Abs7/1
  [VTQR_FEDUWhlTqReqSmoothDelay_Nm] -> VTQR_SPORTFEDUTs_c/1(VTQR_FEDUWhlTqReqSmoothDelay_Nm)
  Abs6/1 -> VTQR_SPORTFEDUTs_c/2(VTQD_TqTargetShaftSpd_rpm)  "VTQD_TqTargetShaftSpd_rpm"
  VTQR_SPORTFEDUTs_c/1(VTQR_SPORTFEDUTs_c) -> Merge/4
  Logical Operator3/1 -> Logical Operator2/2
  [VTQR_FEDUWhlTqReqSmoothDelay_Nm] -> VTQR_NORMALFEDUTs_c/1(VTQR_FEDUWhlTqReqSmoothDelay_Nm)
  Abs8/1 -> VTQR_NORMALFEDUTs_c/2(VTQD_TqTargetShaftSpd_rpm)  "VTQD_TqTargetShaftSpd_rpm"
  VTQR_NORMALFEDUTs_c/1(VTQR_NORMALFEDUTs_c) -> Merge/2
  VTQR_LHMFEDUTs_c/1(VTQR_LHMFEDUTs_c) -> Merge/1
  Equal11/1 -> If/2
  If/1 -> VTQR_LHMFEDUTs_c/Action
  [VTQR_FEDUWhlTqReqSmoothDelay_Nm] -> VTQR_LHMFEDUTs_c/1(VTQR_FEDUWhlTqReqSmoothDelay_Nm)
  Abs5/1 -> VTQR_LHMFEDUTs_c/2(VTQD_TqTargetShaftSpd_rpm)  "VTQD_TqTargetShaftSpd_rpm"
  VTQR_ECOFEDUTs_c/1(VTQR_ECOFEDUTs_c) -> Merge/3
  [VTQR_FEDUWhlTqReqSmoothDelay_Nm] -> VTQR_ECOFEDUTs_c/1(VTQR_FEDUWhlTqReqSmoothDelay_Nm)
  Abs7/1 -> VTQR_ECOFEDUTs_c/2(VTQD_TqTargetShaftSpd_rpm)  "VTQD_TqTargetShaftSpd_rpm"
  VTQD_TqTargetShaftSpd_rpm/1 -> [VTQD_TqTargetShaftSpd_rpm]
  VTQR_EVDriveMode_enum/1 -> [VTQR_EVDriveMode_enum]
  VTQD_RollRegenEnable_flg/1 -> [VTQD_RollRegenEnable_flg]
  VTQD_TqSourceFr_enum/1 -> [VTQD_TqSourceFr_enum]
  VTQR_FEDUWhlTqReqSmoothDelay_Nm/1 -> [VTQR_FEDUWhlTqReqSmoothDelay_Nm]
  VDHP_ActAPSPosn_pct/1 -> [VDHP_ActAPSPosn_pct]
  VINP_VehSpeed_kph/1 -> [VINP_VehSpeed_kph]
  VTQD_LimpHomeAct_flg/1 -> [VTQD_LimpHomeAct_flg]
  VTQD_EVDriveModeValid_flg/1 -> [VTQD_EVDriveModeValid_flg]
  [VTQD_RegenMode_enum] -> VTQR_NORMALFEDUTs_c/3(VTQD_RegenMode_enum)
  [VTQD_RegenMode_enum] -> VTQR_ECOFEDUTs_c/3(VTQD_RegenMode_enum)
  [VTQD_RegenMode_enum] -> VTQR_SPORTFEDUTs_c/3(VTQD_RegenMode_enum)
  If/2 -> VTQR_NORMALFEDUTs_c/Action
  If/3 -> VTQR_ECOFEDUTs_c/Action
  If/4 -> VTQR_SPORTFEDUTs_c/Action
  [VTQD_RollRegenEnable_flg] -> VTQR_ECOFEDUTs_c/4(VTQD_RollRegenEnable_flg)
  VTQD_RegenMode_enum/1 -> [VTQD_RegenMode_enum]
  Abs41/1 -> MTQR_VMCFEDUTs_Z_c/2
  [VTQR_FEDUWhlTqReqSmoothDelay_Nm] -> MTQR_VMCFEDUTs_Z_c/1
  [VVMC_CCPedalOvrd_flg] -> NOT1/1
  Switch2/1 -> VTQR_FrFirstOrderInpTs_c/1  "VTQR_FrFirstOrderInpTs_c"
  NOT/1 -> AND1/2
  NOT1/1 -> AND1/3
  [VTQD_CreepPrLoadEnable_flg] -> Logical Operator14/4
  [VVMC_ACCPedalOvrd_flg] -> NOT/1
  AND1/1 -> Switch3/2
  [VTQD_TqSourceFr_enum] -> Relational Operator1/1
  [VTQR_FEDUTIPOutTs_c] -> Switch13/1
  Constant1/1 -> Relational Operator1/2
  AND2/1 -> Switch13/2
  [VINP_VehSpeed_kph] -> GreaterThan2/1
  Constant34/1 -> Relational Operator4/2
  Constant32/1 -> Less Than2/2
  Relational Operator4/1 -> Logical Operator14/2
  [VDHP_ActAPSPosn_pct] -> Less Than2/1
  [VTQD_TqSourceFr_enum] -> Relational Operator3/1
  Less Than2/1 -> AND2/1
  Constant3/1 -> Relational Operator3/2
  Switch13/1 -> Switch3/3
  Constant33/1 -> GreaterThan2/2
  Logical Operator14/1 -> AND1/1
  Relational Operator3/1 -> Logical Operator14/1
  Relational Operator1/1 -> AND2/3
  [VTQD_TqSourceFr_enum] -> Relational Operator4/1
  GreaterThan2/1 -> AND2/2
  VVMC_ACCPedalOvrd_flg/1 -> [VVMC_ACCPedalOvrd_flg]
  VVMC_CCPedalOvrd_flg/1 -> [VVMC_CCPedalOvrd_flg]
  VTQD_PreLoadHold_flg/1 -> [VTQD_PreLoadHold_flg]
  Switch/1 -> Switch13/3
  Constant4/1 -> Switch/1
  [VTQR_VMCFEDUTs_c] -> Switch1/3
  [VTQD_CreepPrLoadEnable_flg] -> Switch1/2
  Switch1/1 -> Switch3/1
  [VTQR_CreepFEDUTs_c] -> Switch1/1
  VTQD_CreepPrLoadEnable_flg/1 -> [VTQD_CreepPrLoadEnable_flg]
  MTQR_CreepFEDUTs_Z_c/1 -> [VTQR_CreepFEDUTs_c]
  [VTQR_FEDUWhlTqReqSmoothDelay_Nm] -> MTQR_CreepFEDUTs_Z_c/1
  Abs1/1 -> MTQR_CreepFEDUTs_Z_c/2
  [VTQD_TqTargetShaftSpd_rpm] -> Abs1/1
  VTQD_RDCActive_enum/1 -> [VTQD_RDCActive_enum]
  VTQR_NoABSFEDUWhlTqReq_Nm/1 -> [VTQR_NoABSFEDUWhlTqReq_Nm]
  VTQR_RampFEDUWhlTqReq_Nm/1 -> [VTQR_RampFEDUWhlTqReq_Nm]
  Constant5/1 -> Relational Operator2/2
  Relational Operator2/1 -> AND/1
  AND/1 -> [VTQR_FrRDCActiveTs_flg]  "VTQR_FrRDCActiveTs_flg"
  [VTQR_RDCActiveFEDUTs_c] -> Switch2/1
  [VTQD_RDCActive_enum] -> Equal2/1
  Equal2/1 -> AND/2
  [VTQR_FrRDCActiveTs_flg] -> Switch2/2
  Constant7/1 -> Equal2/2
  [VTQR_RampFEDUWhlTqReq_Nm] -> Relational Operator2/1
  Switch3/1 -> Switch2/3
  VTQR_FrFirstOrderInpTq_Nm/1 -> [VTQR_FrFirstOrderInpTq_Nm]
  [VTQR_FrFirstOrderInpTq_Nm] -> Add/2
  OR2/1 -> [VTQR_FrDrModChangeReset_flg]
  Merge/1 -> Switch4/3
  [VTQR_FrDrModTsLatch_flg] -> Delay2/1
  AND4/1 -> OR2/2
  Relational Operator6/1 -> AND4/1
  Delay/1 -> Switch4/1
  Delay2/1 -> AND4/2
  [VTQR_FrDrModChangeReset_flg] -> SR_Latch1/2
  SR_Latch1/1 -> Switch4/2, [VTQR_FrDrModTsLatch_flg]  "VTQR_FrDrModLatch_flg"
  [VTQR_FrFirstOrderInpTq_Nm] -> Add1/2
  Constant8/1 -> Relational Operator5/2
  Switch4/1 -> [VTQR_FEDUTs_c], Delay/1  "VTQR_FEDUTs_c"
  [VTQR_FrFirstOrderInpTq_Nm] -> Delay1/1
  [VTQR_NoABSFEDUWhlTqReq_Nm] -> Add/1
  Delay1/1 -> Add1/1
  Add/1 -> Abs/1
  Abs4/1 -> Relational Operator6/1
  Detect Change/1 -> SR_Latch1/1
  Constant2/1 -> Relational Operator6/2
  Abs/1 -> Relational Operator5/1
  Relational Operator5/1 -> OR2/1
  [VTQR_EVDriveMode_enum] -> Detect Change/1
  Add1/1 -> Abs4/1
  [VTQD_PreLoadHold_flg] -> Switch/2
  Data Type Conversion/1 -> MTQR_AltRDCActiveFEDUTs_Z_c/1
  [VVMC_ActMaxSlideRate_pct] -> MTQR_AltRDCActiveFEDUTs_Z_c/2
  MTQR_AltRDCActiveFEDUTs_Z_c/1 -> [VTQR_RDCActiveFEDUTs_c]  "VTQR_RDCActiveFEDUTs_c"
  [VTQD_RegenMode_enum] -> Data Type Conversion/1
  VVMC_ActMaxSlideRate_pct/1 -> [VVMC_ActMaxSlideRate_pct]
  VTQD_PedAccTqEn_flg/1 -> Terminator/1
  Switch5/1 -> Switch/3
  [VTQR_FEDUTs_c] -> Switch5/3
  [VTQD_PreLoadPreEn_flg] -> Switch5/2
  Constant6/1 -> Switch5/1
  VTQD_PreLoadPreEn_flg/1 -> [VTQD_PreLoadPreEn_flg]
  Relational Operator7/1 -> AND3/1
  [VTQD_TqSourceFr_enum] -> Relational Operator7/1
  VVMC_MSAWhlTqActive_flg/1 -> [VVMC_MSAWhlTqActive_flg]
  [VVMC_MSAWhlTqActive_flg] -> AND3/2
  Constant9/1 -> Relational Operator7/2
  AND3/1 -> Logical Operator14/3

== system tqr/TQR/Determine Torque Request/TorqueArbitrament/TorqueSmooth/Front Torque zero point transfer boundary map ==
  VTQD_TqTargetShaftSpd_rpm : Inport
  VTQR_EVDriveMode_enum : Inport  Port=2
  Constant1 : Constant  Value=ENUM_DRIVEMODE_ECO
  Constant11 : Constant  Value=ENUM_DRIVEMODE_ECO
  Constant12 : Constant  Value=ENUM_DRIVEMODE_NRM
  Constant16 : Constant  Value=ENUM_DRIVEMODE_SPORT
  Constant2 : Constant  Value=ENUM_DRIVEMODE_NRM
  Constant3 : Constant  Value=ENUM_DRIVEMODE_SPORT
  EcoLow : Subsystem  AncestorBlock=tqr/TQR/Determine Torque Request/TorqueArbitrament/TorqueSmooth/Subsystem/EcoUP
  EcoUP : Subsystem
  Equal{1..5,11} (6 alike) : RelationalOperator  Operator===  OutDataTypeStr=boolean  RndMeth=Simplest
  If1 : If  NumInputs=3  IfExpression=u1~= 0  ElseIfExpressions=u2 ~= 0, u3 ~=0  ShowElse=off
  If2 : If  NumInputs=3  IfExpression=u1~= 0  ElseIfExpressions=u2 ~= 0, u3 ~=0  ShowElse=off
  Merge : Merge  Inputs=3
  Merge1 : Merge  Inputs=3
  NormalLow : Subsystem
  NormalUP : Subsystem
  SportLow : Subsystem  AncestorBlock=tqr/TQR/Determine Torque Request/TorqueArbitrament/TorqueSmooth/Subsystem/SportUP
  SportUP : Subsystem
  VTQR_FrTqZeroTransUpBound_Nm : Outport
  VTQR_FrTqZeroTransLowBound_Nm : Outport  Port=2
  wires:
  VTQD_TqTargetShaftSpd_rpm/1 -> [VTQD_TqTargetShaftSpd_rpm]
  VTQR_EVDriveMode_enum/1 -> [VTQR_EVDriveMode_enum]
  Equal11/1 -> If1/1
  [VTQR_EVDriveMode_enum] -> Equal11/1
  Constant12/1 -> Equal11/2
  [VTQR_EVDriveMode_enum] -> Equal1/1
  [VTQR_EVDriveMode_enum] -> Equal2/1
  Equal2/1 -> If1/3
  Constant16/1 -> Equal2/2
  Equal1/1 -> If1/2
  Constant11/1 -> Equal1/2
  [VTQD_TqTargetShaftSpd_rpm] -> NormalUP/1(VTQD_TqTargetShaftSpd_rpm)
  If1/1 -> NormalUP/Action
  If1/2 -> EcoUP/Action
  If1/3 -> SportUP/Action
  [VTQD_TqTargetShaftSpd_rpm] -> EcoUP/1(VTQD_TqTargetShaftSpd_rpm)
  [VTQD_TqTargetShaftSpd_rpm] -> SportUP/1(VTQD_TqTargetShaftSpd_rpm)
  NormalUP/1(VTQR_FrTqZeroTransUpBound_Nm) -> Merge/1
  EcoUP/1(VTQR_FrTqZeroTransUpBound_Nm) -> Merge/2
  SportUP/1(VTQR_FrTqZeroTransUpBound_Nm) -> Merge/3
  [VTQD_TqTargetShaftSpd_rpm] -> NormalLow/1(VTQD_TqTargetShaftSpd_rpm)
  EcoLow/1(VTQR_FrTqZeroTransLowBound_Nm) -> Merge1/2
  SportLow/1(VTQR_FrTqZeroTransLowBound_Nm) -> Merge1/3
  [VTQD_TqTargetShaftSpd_rpm] -> SportLow/1(VTQD_TqTargetShaftSpd_rpm)
  Constant3/1 -> Equal5/2
  Equal3/1 -> If2/2
  Merge1/1 -> VTQR_FrTqZeroTransLowBound_Nm/1  "VTQR_FrTqZeroTransLowBound_Nm"
  Equal4/1 -> If2/1
  Constant1/1 -> Equal3/2
  [VTQR_EVDriveMode_enum] -> Equal5/1
  [VTQR_EVDriveMode_enum] -> Equal3/1
  [VTQR_EVDriveMode_enum] -> Equal4/1
  [VTQD_TqTargetShaftSpd_rpm] -> EcoLow/1(VTQD_TqTargetShaftSpd_rpm)
  NormalLow/1(VTQR_FrTqZeroTransLowBound_Nm) -> Merge1/1
  Constant2/1 -> Equal4/2
  Equal5/1 -> If2/3
  Merge/1 -> VTQR_FrTqZeroTransUpBound_Nm/1  "VTQR_FrTqZeroTransUpBound_Nm"
  If2/1 -> NormalLow/Action
  If2/2 -> EcoLow/Action
  If2/3 -> SportLow/Action
